simulink model "ModelMotS_dq_V2bis_FVC"  (R2019b)
settings: Solver=ode45  StartTime=0.0  StopTime=10  MaxStep=1e-4  RelTol=1e-4  EnableMultiTasking=on
undefined symbols (not defined in the file): Data_Ts, DiscIntNeverNeededParam, Inom, J, Jm, Lfr, Lfs, Lm, Lmt, Lr, Ls, np, P1, P2, Prdnom, Prinit, Psinit, Rr, Rs, SFC_Coeff, SLP_Coeff, thrinit, Tpwm, Vnom, wCurr, wCurr_PI, wL, wrinit, wSpeed_PI, wSpeedEst, xiCurr_PI, xiSpeed_PI
libraries: simulink x5
settings Model: Creator=stbp106  LastModifiedBy=versag
settings DataIOCC: LimitDataPoints=on  SaveFormat=Array  ReturnWorkspaceOutputs=off
settings OptimizationCC: LifeSpan=inf
settings DebuggingCC: UnderspecifiedInitializationDetection=Classic  MergeDetectMultiDrivingBlocksExec=none  SolverPrmCheckMsg=warning  SFUnexpectedBacktrackingDiag=warning  SFNoUnconditionalDefaultTransitionDiag=warning  SFExecutionAtInitializationDiag=none  ArithmeticOperatorsInVariantConditions=warning
settings HardwareCC: ProdBitPerPointer=32  ProdBitPerSizeT=32  ProdBitPerPtrDiffT=32  ProdLargestAtomicFloat=None  ProdIntDivRoundTo=Undefined  ProdEndianess=Unspecified  ProdWordSize=32  ProdHWDeviceType=32-bit Generic
settings ModelReferenceCC: PropagateSignalLabelsOutOfModel=off
settings SFSimCC: SimUseLocalCustomCode=off  CustomCodeUndefinedFunction=UseInterfaceOnly
settings RTWCC: RTWUseLocalCustomCode=off
settings CodeAppCC: StateflowObjectComments=on
settings GRTTargetCC: TargetLangStandard=C89/C90 (ANSI)  GeneratePreprocessorConditionals=Disable all
settings ConfigComp: CovMetricSettings=dw  CovHtmlReporting=on  CovSaveCumulativeToWorkspaceVar=on  CovSaveSingleToWorkspaceVar=on  CovExternalEMLEnable=off  CovSFcnEnable=off

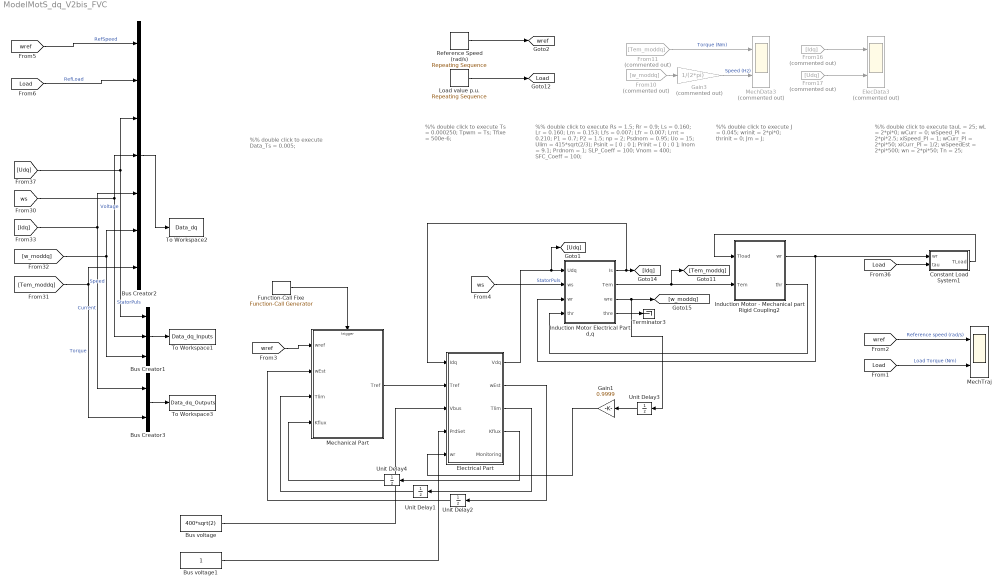
== system ModelMotS_dq_V2bis_FVC ==
  note: %% double click to execute
      |
      | Rs = 1.5; Rr = 0.9;
      | Ls = 0.160; Lr = 0.160; Lm = 0.153;
      | Lfs = 0.007; Lfr = 0.007; Lmt = 0.210; P1 = 0.7; P2 = 1.5;
      | np = 2;
      | Psdnom = 0.95; Uo = 15; Ulim = 415*sqrt(2/3);
      | Psinit = [ 0 ; 0 ]; Prinit = [ 0 ; 0 ];
      | Inom = 9.1; Prdnom = 1; SLP_Coeff = 100; Vnom = 400;
      | SFC_Coeff = 100;
  note: %% double click to execute
      |
      | J = 0.045;
      | wrinit = 2*pi*0;
      | thrinit = 0;
      | Jm = J;
  note: %% double click to execute
      |
      | tauL = 25;
      | wL = 2*pi*0;
      |
      | wCurr = 0;
      | wSpeed_PI = 2*pi*2.5; xiSpeed_PI = 1;
      | wCurr_PI = 2*pi*50; xiCurr_PI = 1/2;
      | wSpeedEst = 2*pi*500;
      |
      | wn = 2*pi*50;
      | Tn = 25;
  note: %% double click to execute
      |
      | Ts = 0.000250;
      | Tpwm = Ts;
      | Tfixe = 500e-6;
  note: %% double click to execute
      |
      | Data_Ts = 0.005;
  Bus Creator1 : BusCreator  Inputs=3
  Bus Creator2 : BusCreator  Inputs=7
  Bus Creator3 : BusCreator  Inputs=2
  Bus voltage : Constant  Value=400*sqrt(2)
  Bus voltage1 : Constant
  Constant Load System1 : Subsystem  Description=""
  ElecData3 : Scope  Commented=on  NumInputPorts=2
  Electrical Part : Subsystem
  From10 : From  Commented=on  GotoTag=w_moddq
  From11 : From  Commented=on  GotoTag=Tem_moddq
  From16 : From  Commented=on  GotoTag=Idq
  From17 : From  Commented=on  GotoTag=Udq
  Function-Call Fixe : simulink/Ports & Subsystems/Function-Call Generator  sample_time=Tfixe  numberOfIterations=1
  Gain1 : Gain  Gain=0.9999
  Gain3 : Gain  Commented=on  Gain=1/(2*pi)  SaturateOnIntegerOverflow=on  OutDataTypeStr=Inherit: Same as input  ParamDataTypeStr=Inherit: Same as input
  Induction Motor Electrical Part d,q : Subsystem  Description=""
  Induction Motor - Mechanical part Rigid Coupling2 : Subsystem  Description=""
  Load value p.u. : simulink/Sources/Repeating Sequence  rep_seq_t=[0 1 2.5 4 5.5 7 8.5 10]  rep_seq_y=[0 0 0 0 0 0 0 0] / 100 * 25
  MechData3 : Scope  Commented=on  NumInputPorts=2
  MechTraj : Scope  NumInputPorts=2
  Mechanical Part : Subsystem
  Reference Speed (rad/s) : simulink/Sources/Repeating Sequence  rep_seq_t=[0 1 2.5 4 5.5 7 8.5 10]  rep_seq_y=[0 0 50 50 -50 -50 25 25]*2*pi
  Terminator3 : Terminator
  To Workspace1 : ToWorkspace  VariableName=Data_dq_Inputs  SaveFormat=Timeseries  SampleTime=Data_Ts
  To Workspace2 : ToWorkspace  VariableName=Data_dq  SaveFormat=Timeseries  SampleTime=Data_Ts
  To Workspace3 : ToWorkspace  VariableName=Data_dq_Outputs  SaveFormat=Timeseries  SampleTime=Data_Ts
  Unit Delay{1..4} (4 alike) : UnitDelay  SampleTime=-1  HasFrameUpgradeWarning=on
  tag scope: Load=global, wref=global
  wires:
  Reference Speed (rad/s)/1 -> [wref]
  Induction Motor - Mechanical part Rigid Coupling2/2(thr) -> Induction Motor Electrical Part d,q/4(thr)
  Induction Motor Electrical Part d,q/2(Tem) -> [Tem_moddq], Induction Motor - Mechanical part Rigid Coupling2/2(Tem)
  Induction Motor - Mechanical part Rigid Coupling2/1(wr) -> Constant Load System1/1(wr), Induction Motor Electrical Part d,q/3(wr)
  Induction Motor Electrical Part d,q/4(thre) -> Terminator3/1
  Constant Load System1/1(TLoad) -> Induction Motor - Mechanical part Rigid Coupling2/1(Tload)
  Induction Motor Electrical Part d,q/1(Is) -> Electrical Part/1(Idq), [Idq]
  Induction Motor Electrical Part d,q/3(wre) -> Unit Delay3/1, [w_moddq]
  [Load] -> Constant Load System1/2(tau)
  From16/1 -> ElecData3/1
  From17/1 -> ElecData3/2
  From10/1 -> Gain3/1
  From11/1 -> MechData3/1  "Torque (Nm)"
  Gain3/1 -> MechData3/2  "Speed (Hz)"
  Load value p.u./1 -> [Load]
  [Udq] -> Bus Creator1/1, Bus Creator2/3  "Voltage"
  [Idq] -> Bus Creator3/1, Bus Creator2/5  "Current"
  [w_moddq] -> Bus Creator1/3, Bus Creator2/6  "Speed"
  [Tem_moddq] -> Bus Creator3/2, Bus Creator2/7  "Torque"
  Bus Creator2/1 -> To Workspace2/1
  [ws] -> Bus Creator1/2, Bus Creator2/4  "StatorPuls"
  [Load] -> MechTraj/2  "Load Torque (Nm)"
  [wref] -> MechTraj/1  "Reference speed (rad/s)"
  Mechanical Part/1(Tref) -> Electrical Part/2(Tref)
  [wref] -> Mechanical Part/1(wref)
  Electrical Part/2(wEst) -> Unit Delay2/1
  Electrical Part/3(Tlim) -> Unit Delay1/1
  Electrical Part/4(Kflux) -> Unit Delay4/1
  Unit Delay4/1 -> Mechanical Part/4(Kflux)
  Unit Delay1/1 -> Mechanical Part/3(Tlim)
  Unit Delay2/1 -> Mechanical Part/2(wEst)
  Electrical Part/1(Vdq) -> [Udq], Induction Motor Electrical Part d,q/1(Udq)
  [ws] -> Induction Motor Electrical Part d,q/2(ws)  "StatorPuls"
  Unit Delay3/1 -> Gain1/1
  Gain1/1 -> Electrical Part/5(wr)
  Bus voltage/1 -> Electrical Part/3(Vbus)
  Bus voltage1/1 -> Electrical Part/4(PrdSet)
  Function-Call Fixe/1 -> Mechanical Part/Trigger
  Bus Creator3/1 -> To Workspace3/1
  Bus Creator1/1 -> To Workspace1/1
  [wref] -> Bus Creator2/1  "RefSpeed"
  [Load] -> Bus Creator2/2  "RefLoad"

== system ModelMotS_dq_V2bis_FVC/Constant Load System1 ==
  wr : Inport
  tau : Inport  Port=2
  Constant1 : Constant  Value=wL
  Fcn : Fcn  Expr=u(1)/sqrt( u(1)^2 + (2*pi*0.1)^2)
  Product2 : Product  RndMeth=Zero
  Sum2 : Sum  Inputs=+-  SaturateOnIntegerOverflow=on  InputSameDT=on  OutDataTypeStr=Inherit: Same as first input
  TLoad : Outport  VectorParamsAs1DForOutWhenUnconnected=off
  wires:
  Product2/1 -> TLoad/1
  wr/1 -> Sum2/1
  Constant1/1 -> Sum2/2
  Sum2/1 -> Fcn/1
  Fcn/1 -> Product2/1
  tau/1 -> Product2/2

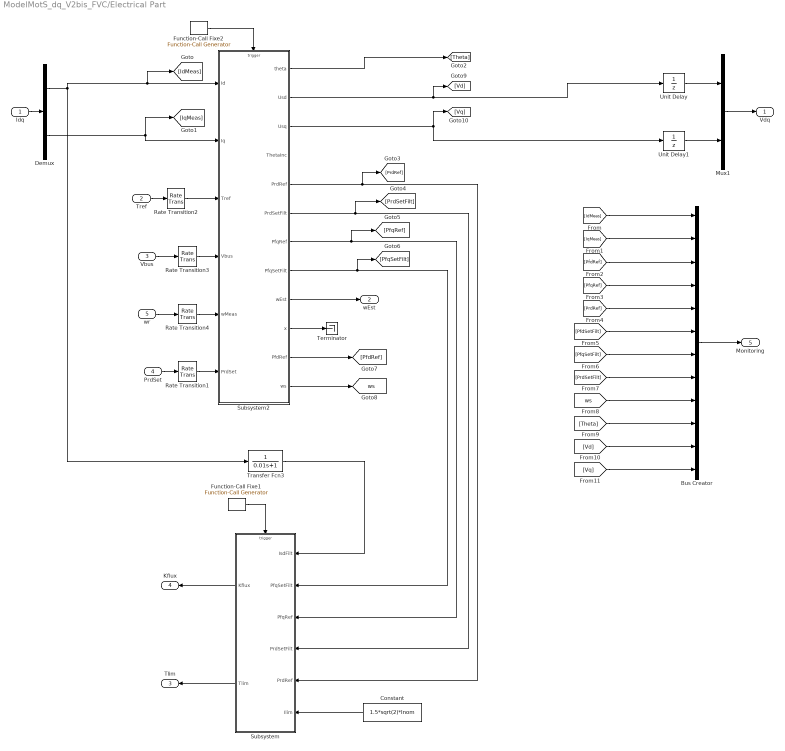
== system ModelMotS_dq_V2bis_FVC/Electrical Part ==
  Idq : Inport
  Tref : Inport  Port=2
  Vbus : Inport  Port=3
  PrdSet : Inport  Port=4
  wr : Inport  Port=5
  Bus Creator : BusCreator  Inputs=12
  Constant : Constant  Value=1.5*sqrt(2)*Inom
  Demux : Demux  Outputs=2
  Function-Call Fixe1 : simulink/Ports & Subsystems/Function-Call Generator  sample_time=Ts  numberOfIterations=1
  Function-Call Fixe2 : simulink/Ports & Subsystems/Function-Call Generator  sample_time=Ts  numberOfIterations=1
  Mux1 : Mux  Inputs=2
  Rate Transition{1..4} (4 alike) : RateTransition
  Subsystem : Subsystem
  Subsystem2 : Subsystem
  Terminator : Terminator
  Transfer Fcn3 : TransferFcn  Denominator=[0.01 1]
  Unit Delay : UnitDelay  SampleTime=-1  HasFrameUpgradeWarning=on
  Unit Delay1 : UnitDelay  SampleTime=-1  HasFrameUpgradeWarning=on
  Vdq : Outport  VectorParamsAs1DForOutWhenUnconnected=off
  wEst : Outport  Port=2  VectorParamsAs1DForOutWhenUnconnected=off
  Tlim : Outport  Port=3  VectorParamsAs1DForOutWhenUnconnected=off
  Kflux : Outport  Port=4  VectorParamsAs1DForOutWhenUnconnected=off
  Monitoring : Outport  Port=5  VectorParamsAs1DForOutWhenUnconnected=off
  tag scope: ws=global
  wires:
  [IqMeas] -> Bus Creator/2
  [IdMeas] -> Bus Creator/1
  [PfdRef] -> Bus Creator/3
  [PfqRef] -> Bus Creator/4
  [PrdRef] -> Bus Creator/5
  [PrdSetFilt] -> Bus Creator/8
  [PfqSetFilt] -> Bus Creator/7
  [PfdSetFilt] -> Bus Creator/6
  [ws] -> Bus Creator/9
  [Theta] -> Bus Creator/10
  Bus Creator/1 -> Monitoring/1
  Transfer Fcn3/1 -> Subsystem/1(IsdFilt)
  Subsystem/1(Kflux) -> Kflux/1
  Subsystem/2(Tlim) -> Tlim/1
  [Vd] -> Bus Creator/11
  [Vq] -> Bus Creator/12
  Subsystem2/7(PfqRef) -> [PfqRef], Subsystem/3(PfqRef)
  Subsystem2/6(PrdSetFilt) -> [PrdSetFilt], Subsystem/4(PrdSetFilt)
  Subsystem2/8(PfqSetFilt) -> [PfqSetFilt], Subsystem/2(PfqSetFilt)
  Subsystem2/1(theta) -> [Theta]
  Subsystem2/5(PrdRef) -> [PrdRef], Subsystem/5(PrdRef)
  Tref/1 -> Rate Transition2/1
  Vbus/1 -> Rate Transition3/1
  wr/1 -> Rate Transition4/1
  Subsystem2/9(wEst) -> wEst/1
  Subsystem2/11(PfdRef) -> [PfdRef]
  Subsystem2/12(ws) -> [ws]
  Demux/2 -> [IqMeas], Subsystem2/2(Iq)
  Demux/1 -> Subsystem2/1(Id), [IdMeas], Transfer Fcn3/1
  Function-Call Fixe2/1 -> Subsystem2/Trigger
  Function-Call Fixe1/1 -> Subsystem/Trigger
  Rate Transition2/1 -> Subsystem2/3(Tref)
  Subsystem2/10(x) -> Terminator/1
  Constant/1 -> Subsystem/6(Ilim)
  Rate Transition3/1 -> Subsystem2/4(Vbus)
  Rate Transition4/1 -> Subsystem2/5(wMeas)
  Mux1/1 -> Vdq/1
  PrdSet/1 -> Rate Transition1/1
  Rate Transition1/1 -> Subsystem2/6(PrdSet)
  Subsystem2/3(Usq) -> Unit Delay1/1, [Vq]
  Subsystem2/2(Usd) -> Unit Delay/1, [Vd]
  Unit Delay/1 -> Mux1/1
  Unit Delay1/1 -> Mux1/2
  Idq/1 -> Demux/1

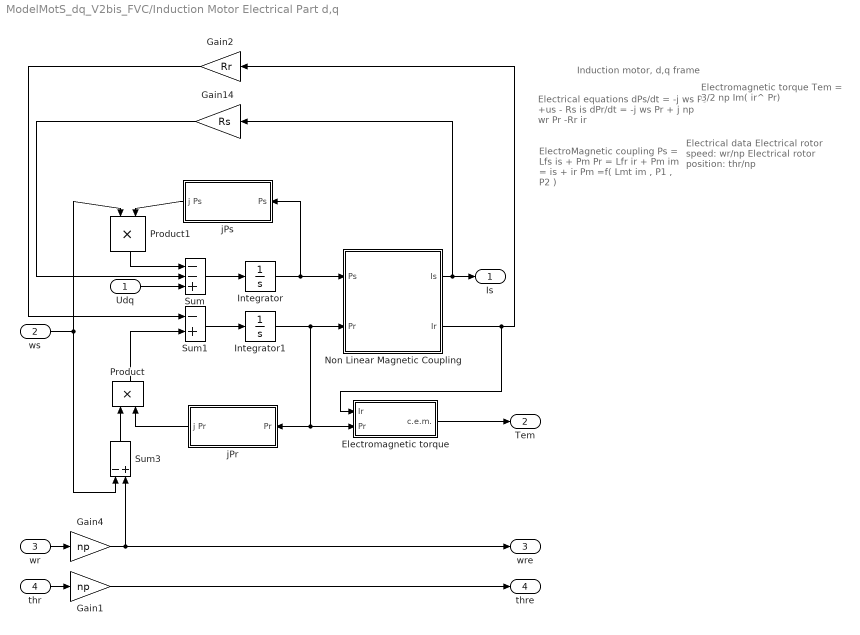
== system ModelMotS_dq_V2bis_FVC/Induction Motor Electrical Part d,q ==
  note: Electrical equations
      | dPs/dt =  -j ws Ps +us - Rs is
      | dPr/dt = -j ws Pr + j np wr Pr -Rr ir
  note: Electromagnetic torque
      | Tem = 3/2 np Im( ir^ Pr)
  note: Induction motor, d,q frame
  note: Electrical data
      | Electrical rotor speed: wr/np
      | Electrical rotor position: thr/np
  note: ElectroMagnetic coupling
      | Ps  = Lfs is + Pm
      | Pr  = Lfr ir + Pm
      |
      | im = is + ir
      | Pm =f( Lmt im , P1 , P2 )
  Udq : Inport
  ws : Inport  Port=2
  wr : Inport  Port=3
  thr : Inport  Port=4
  Electromagnetic torque : Subsystem
  Gain1 : Gain  Gain=np  SaturateOnIntegerOverflow=on  OutDataTypeStr=Inherit: Same as input  ParamDataTypeStr=Inherit: Same as input
  Gain14 : Gain  Gain=Rs  SaturateOnIntegerOverflow=on  OutDataTypeStr=Inherit: Same as input  ParamDataTypeStr=Inherit: Same as input
  Gain2 : Gain  Gain=Rr  SaturateOnIntegerOverflow=on  OutDataTypeStr=Inherit: Same as input  ParamDataTypeStr=Inherit: Same as input
  Gain4 : Gain  Gain=np  SaturateOnIntegerOverflow=on  OutDataTypeStr=Inherit: Same as input  ParamDataTypeStr=Inherit: Same as input
  Integrator : Integrator  InitialCondition=Psinit
  Integrator1 : Integrator  InitialCondition=Prinit
  Non Linear Magnetic Coupling : Subsystem
  Product : Product  SaturateOnIntegerOverflow=on  RndMeth=Zero  InputSameDT=on  OutDataTypeStr=Inherit: Same as first input
  Product1 : Product  SaturateOnIntegerOverflow=on  RndMeth=Zero  InputSameDT=on  OutDataTypeStr=Inherit: Same as first input
  Sum : Sum  Inputs=--+  SaturateOnIntegerOverflow=on  InputSameDT=on  OutDataTypeStr=Inherit: Same as first input
  Sum1 : Sum  Inputs=-+  SaturateOnIntegerOverflow=on  InputSameDT=on  OutDataTypeStr=Inherit: Same as first input
  Sum3 : Sum  Inputs=-+  SaturateOnIntegerOverflow=on  InputSameDT=on  OutDataTypeStr=Inherit: Same as first input
  jPr : Subsystem
  jPs : Subsystem
  Is : Outport  VectorParamsAs1DForOutWhenUnconnected=off
  Tem : Outport  Port=2  VectorParamsAs1DForOutWhenUnconnected=off
  wre : Outport  Port=3  VectorParamsAs1DForOutWhenUnconnected=off
  thre : Outport  Port=4  VectorParamsAs1DForOutWhenUnconnected=off
  wires:
  Integrator1/1 -> Non Linear Magnetic Coupling/2(Pr), Electromagnetic torque/2(Pr), jPr/1(Pr)
  Electromagnetic torque/1(c.e.m.) -> Tem/1
  Non Linear Magnetic Coupling/2(Ir) -> Electromagnetic torque/1(Ir), Gain2/1
  Product/1 -> Sum1/2
  jPr/1(j Pr) -> Product/2
  Gain2/1 -> Sum1/1
  Sum1/1 -> Integrator1/1
  Non Linear Magnetic Coupling/1(Is) -> Is/1, Gain14/1
  Sum/1 -> Integrator/1
  Udq/1 -> Sum/3
  Gain14/1 -> Sum/2
  jPs/1(j Ps) -> Product1/2
  Product1/1 -> Sum/1
  Integrator/1 -> Non Linear Magnetic Coupling/1(Ps), jPs/1(Ps)
  Sum3/1 -> Product/1
  Gain4/1 -> wre/1, Sum3/2
  ws/1 -> Product1/1, Sum3/1
  wr/1 -> Gain4/1
  thr/1 -> Gain1/1
  Gain1/1 -> thre/1

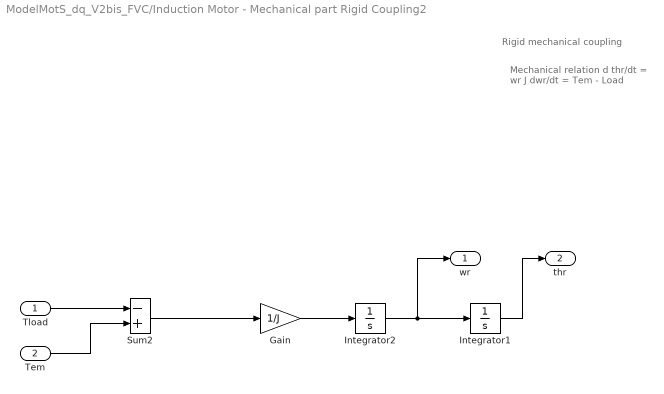
== system ModelMotS_dq_V2bis_FVC/Induction Motor - Mechanical part Rigid Coupling2 ==
  note: Rigid mechanical coupling
  note: Mechanical relation
      | d thr/dt = wr
      | J dwr/dt = Tem - Load
  Tload : Inport
  Tem : Inport  Port=2
  Gain : Gain  Gain=1/J  SaturateOnIntegerOverflow=on  OutDataTypeStr=Inherit: Same as input  ParamDataTypeStr=Inherit: Same as input
  Integrator1 : Integrator  InitialCondition=thrinit
  Integrator2 : Integrator  InitialCondition=wrinit
  Sum2 : Sum  Inputs=-+  SaturateOnIntegerOverflow=on  InputSameDT=on  OutDataTypeStr=Inherit: Same as first input
  wr : Outport  VectorParamsAs1DForOutWhenUnconnected=off
  thr : Outport  Port=2  VectorParamsAs1DForOutWhenUnconnected=off
  wires:
  Integrator1/1 -> thr/1
  Integrator2/1 -> wr/1, Integrator1/1
  Tem/1 -> Sum2/2
  Tload/1 -> Sum2/1
  Gain/1 -> Integrator2/1
  Sum2/1 -> Gain/1

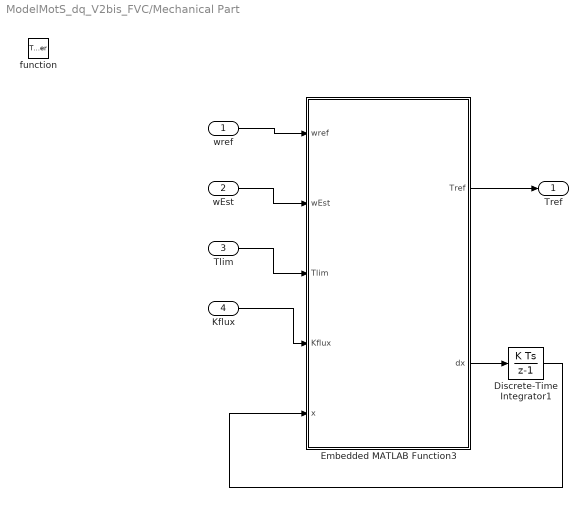
== system ModelMotS_dq_V2bis_FVC/Mechanical Part ==
  wref : Inport
  wEst : Inport  Port=2
  Tlim : Inport  Port=3
  Kflux : Inport  Port=4
  function : TriggerPort  TriggerType=function-call  VariantControl=(inherit)
  Discrete-Time Integrator1 : DiscreteIntegrator  InitialCondition=zeros(1,2)  SampleTime=-1  ICPrevOutput=DiscIntNeverNeededParam  ICPrevScaledInput=DiscIntNeverNeededParam
  Embedded MATLAB Function3 : MATLAB Function  TreatAsAtomicUnit=on
  Tref : Outport  VectorParamsAs1DForOutWhenUnconnected=off
  wires:
  Discrete-Time Integrator1/1 -> Embedded MATLAB Function3/5(x)
  wEst/1 -> Embedded MATLAB Function3/2(wEst)
  Tlim/1 -> Embedded MATLAB Function3/3(Tlim)
  wref/1 -> Embedded MATLAB Function3/1(wref)
  Embedded MATLAB Function3/2(dx) -> Discrete-Time Integrator1/1
  Embedded MATLAB Function3/1(Tref) -> Tref/1
  Kflux/1 -> Embedded MATLAB Function3/4(Kflux)

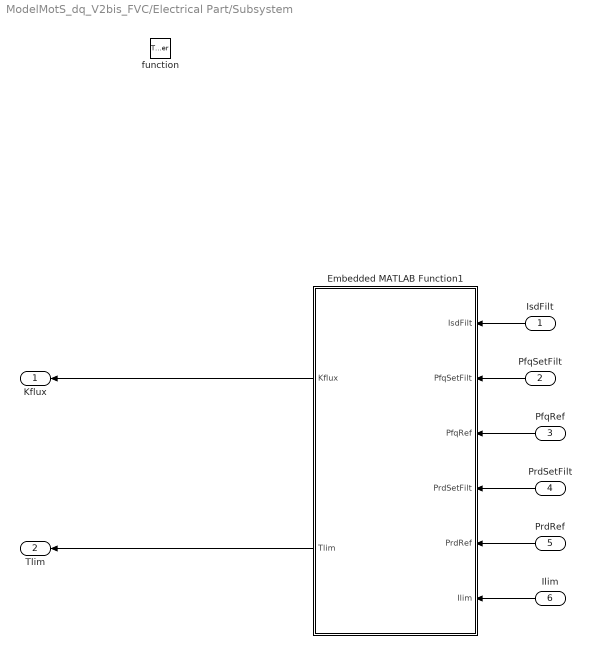
== system ModelMotS_dq_V2bis_FVC/Electrical Part/Subsystem ==
  IsdFilt : Inport
  PfqSetFilt : Inport  Port=2
  PfqRef : Inport  Port=3
  PrdSetFilt : Inport  Port=4
  PrdRef : Inport  Port=5
  Ilim : Inport  Port=6
  function : TriggerPort  TriggerType=function-call  VariantControl=(inherit)
  Embedded MATLAB Function1 : MATLAB Function  TreatAsAtomicUnit=on
  Kflux : Outport  VectorParamsAs1DForOutWhenUnconnected=off
  Tlim : Outport  Port=2  VectorParamsAs1DForOutWhenUnconnected=off
  wires:
  Embedded MATLAB Function1/2(Tlim) -> Tlim/1
  IsdFilt/1 -> Embedded MATLAB Function1/1(IsdFilt)
  Embedded MATLAB Function1/1(Kflux) -> Kflux/1
  PrdSetFilt/1 -> Embedded MATLAB Function1/4(PrdSetFilt)
  PfqSetFilt/1 -> Embedded MATLAB Function1/2(PfqSetFilt)
  PfqRef/1 -> Embedded MATLAB Function1/3(PfqRef)
  PrdRef/1 -> Embedded MATLAB Function1/5(PrdRef)
  Ilim/1 -> Embedded MATLAB Function1/6(Ilim)

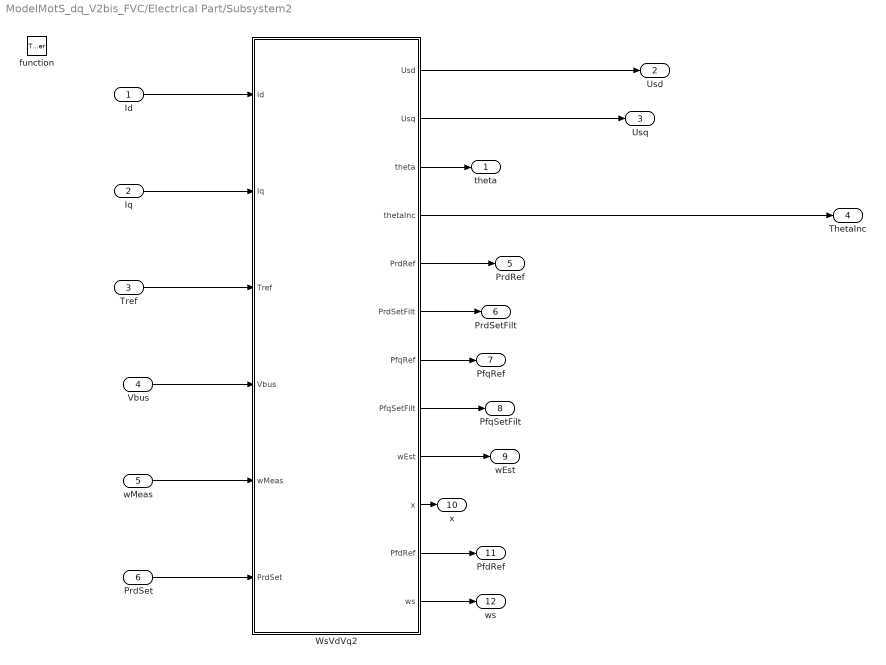
== system ModelMotS_dq_V2bis_FVC/Electrical Part/Subsystem2 ==
  Id : Inport
  Iq : Inport  Port=2
  Tref : Inport  Port=3
  Vbus : Inport  Port=4
  wMeas : Inport  Port=5
  PrdSet : Inport  Port=6
  function : TriggerPort  TriggerType=function-call  VariantControl=(inherit)
  WsVdVq2 : Subsystem
  theta : Outport  VectorParamsAs1DForOutWhenUnconnected=off
  Usd : Outport  Port=2  VectorParamsAs1DForOutWhenUnconnected=off
  Usq : Outport  Port=3  VectorParamsAs1DForOutWhenUnconnected=off
  ThetaInc : Outport  Port=4  VectorParamsAs1DForOutWhenUnconnected=off
  PrdRef : Outport  Port=5  VectorParamsAs1DForOutWhenUnconnected=off
  PrdSetFilt : Outport  Port=6  VectorParamsAs1DForOutWhenUnconnected=off
  PfqRef : Outport  Port=7  VectorParamsAs1DForOutWhenUnconnected=off
  PfqSetFilt : Outport  Port=8  VectorParamsAs1DForOutWhenUnconnected=off
  wEst : Outport  Port=9  VectorParamsAs1DForOutWhenUnconnected=off
  x : Outport  Port=10  VectorParamsAs1DForOutWhenUnconnected=off
  PfdRef : Outport  Port=11  VectorParamsAs1DForOutWhenUnconnected=off
  ws : Outport  Port=12  VectorParamsAs1DForOutWhenUnconnected=off
  wires:
  WsVdVq2/7(PfqRef) -> PfqRef/1
  WsVdVq2/9(wEst) -> wEst/1
  Tref/1 -> WsVdVq2/3(Tref)
  WsVdVq2/8(PfqSetFilt) -> PfqSetFilt/1
  WsVdVq2/6(PrdSetFilt) -> PrdSetFilt/1
  Vbus/1 -> WsVdVq2/4(Vbus)
  wMeas/1 -> WsVdVq2/5(wMeas)
  WsVdVq2/5(PrdRef) -> PrdRef/1
  WsVdVq2/3(theta) -> theta/1
  WsVdVq2/12(ws) -> ws/1
  WsVdVq2/11(PfdRef) -> PfdRef/1
  WsVdVq2/2(Usq) -> Usq/1
  WsVdVq2/4(thetaInc) -> ThetaInc/1
  WsVdVq2/1(Usd) -> Usd/1
  WsVdVq2/10(x) -> x/1
  Id/1 -> WsVdVq2/1(Id)
  Iq/1 -> WsVdVq2/2(Iq)
  PrdSet/1 -> WsVdVq2/6(PrdSet)

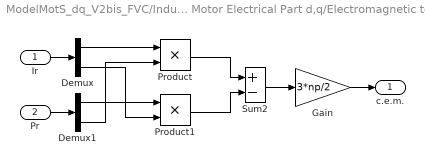
== system ModelMotS_dq_V2bis_FVC/Induction Motor Electrical Part d,q/Electromagnetic torque ==
  Ir : Inport
  Pr : Inport  Port=2
  Demux : Demux  Outputs=2
  Demux1 : Demux  Outputs=2
  Gain : Gain  Gain=3*np/2  SaturateOnIntegerOverflow=on  OutDataTypeStr=Inherit: Same as input  ParamDataTypeStr=Inherit: Same as input
  Product : Product  SaturateOnIntegerOverflow=on  RndMeth=Zero  InputSameDT=on  OutDataTypeStr=Inherit: Same as first input
  Product1 : Product  SaturateOnIntegerOverflow=on  RndMeth=Zero  InputSameDT=on  OutDataTypeStr=Inherit: Same as first input
  Sum2 : Sum  Inputs=+-  SaturateOnIntegerOverflow=on  InputSameDT=on  OutDataTypeStr=Inherit: Same as first input
  c.e.m. : Outport  VectorParamsAs1DForOutWhenUnconnected=off
  wires:
  Pr/1 -> Demux1/1
  Gain/1 -> c.e.m./1
  Ir/1 -> Demux/1
  Demux/2 -> Product1/2
  Demux1/1 -> Product1/1
  Demux1/2 -> Product/2
  Demux/1 -> Product/1
  Sum2/1 -> Gain/1
  Product1/1 -> Sum2/2
  Product/1 -> Sum2/1

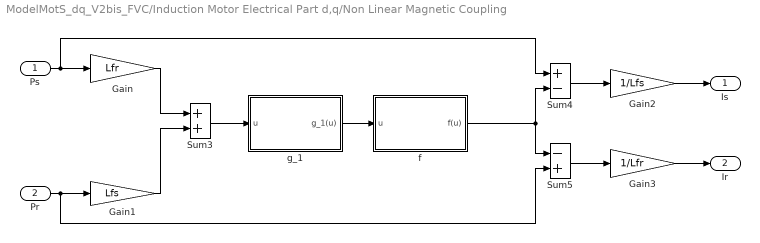
== system ModelMotS_dq_V2bis_FVC/Induction Motor Electrical Part d,q/Non Linear Magnetic Coupling ==
  Ps : Inport
  Pr : Inport  Port=2
  Gain : Gain  Gain=Lfr  SaturateOnIntegerOverflow=on  OutDataTypeStr=Inherit: Same as input  ParamDataTypeStr=Inherit: Same as input
  Gain1 : Gain  Gain=Lfs  SaturateOnIntegerOverflow=on  OutDataTypeStr=Inherit: Same as input  ParamDataTypeStr=Inherit: Same as input
  Gain2 : Gain  Gain=1/Lfs  SaturateOnIntegerOverflow=on  OutDataTypeStr=Inherit: Same as input  ParamDataTypeStr=Inherit: Same as input
  Gain3 : Gain  Gain=1/Lfr  SaturateOnIntegerOverflow=on  OutDataTypeStr=Inherit: Same as input  ParamDataTypeStr=Inherit: Same as input
  Sum3 : Sum  SaturateOnIntegerOverflow=on  InputSameDT=on  OutDataTypeStr=Inherit: Same as first input
  Sum4 : Sum  Inputs=+-  SaturateOnIntegerOverflow=on  InputSameDT=on  OutDataTypeStr=Inherit: Same as first input
  Sum5 : Sum  Inputs=-+  SaturateOnIntegerOverflow=on  InputSameDT=on  OutDataTypeStr=Inherit: Same as first input
  f : Subsystem
  g_1 : Subsystem
  Is : Outport  VectorParamsAs1DForOutWhenUnconnected=off
  Ir : Outport  Port=2  VectorParamsAs1DForOutWhenUnconnected=off
  wires:
  Gain2/1 -> Is/1
  Gain3/1 -> Ir/1
  Sum5/1 -> Gain3/1
  Sum4/1 -> Gain2/1
  Pr/1 -> Sum5/2, Gain1/1
  Ps/1 -> Sum4/1, Gain/1
  f/1(f(u)) -> Sum4/2, Sum5/1
  g_1/1(g_1(u)) -> f/1(u)
  Sum3/1 -> g_1/1(u)
  Gain1/1 -> Sum3/2
  Gain/1 -> Sum3/1

== system ModelMotS_dq_V2bis_FVC/Induction Motor Electrical Part d,q/jPr ==
  Pr : Inport
  Demux1 : Demux  Outputs=2
  Gain : Gain  Gain=-1  SaturateOnIntegerOverflow=on  OutDataTypeStr=Inherit: Same as input  ParamDataTypeStr=Inherit: Same as input
  Mux : Mux  Inputs=2
  j Pr : Outport  VectorParamsAs1DForOutWhenUnconnected=off
  wires:
  Mux/1 -> j Pr/1
  Gain/1 -> Mux/1
  Demux1/2 -> Gain/1
  Demux1/1 -> Mux/2
  Pr/1 -> Demux1/1

== system ModelMotS_dq_V2bis_FVC/Induction Motor Electrical Part d,q/jPs ==
  Ps : Inport
  Demux1 : Demux  Outputs=2
  Gain : Gain  Gain=-1  SaturateOnIntegerOverflow=on  OutDataTypeStr=Inherit: Same as input  ParamDataTypeStr=Inherit: Same as input
  Mux : Mux  Inputs=2
  j Ps : Outport  VectorParamsAs1DForOutWhenUnconnected=off
  wires:
  Ps/1 -> Demux1/1
  Demux1/1 -> Mux/2
  Demux1/2 -> Gain/1
  Gain/1 -> Mux/1
  Mux/1 -> j Ps/1

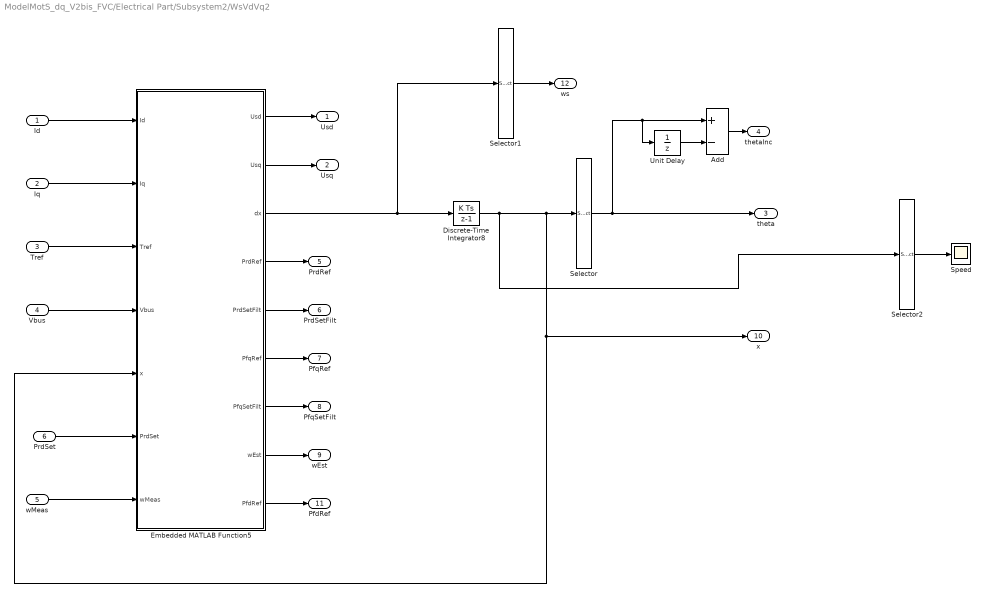
== system ModelMotS_dq_V2bis_FVC/Electrical Part/Subsystem2/WsVdVq2 ==
  Id : Inport
  Iq : Inport  Port=2
  Tref : Inport  Port=3
  Vbus : Inport  Port=4
  wMeas : Inport  Port=5
  PrdSet : Inport  Port=6
  Add : Sum  Inputs=+-
  Discrete-Time Integrator8 : DiscreteIntegrator  InitialCondition=[1/(Lm^2/Lr),0,1,zeros(1,9)]  SampleTime=-1  ICPrevOutput=DiscIntNeverNeededParam  ICPrevScaledInput=DiscIntNeverNeededParam
  Embedded MATLAB Function5 : MATLAB Function  TreatAsAtomicUnit=on
  Selector : Selector  InputPortWidth=12  IndexOptions=Index vector (dialog)  Indices=5  OutputSizes=1
  Selector1 : Selector  InputPortWidth=12  IndexOptions=Index vector (dialog)  Indices=5  OutputSizes=1
  Selector2 : Selector  InputPortWidth=12  IndexOptions=Index vector (dialog)  Indices=[11 12]  OutputSizes=1
  Speed : Scope
  Unit Delay : UnitDelay  SampleTime=-1  HasFrameUpgradeWarning=on
  Usd : Outport  VectorParamsAs1DForOutWhenUnconnected=off
  Usq : Outport  Port=2  VectorParamsAs1DForOutWhenUnconnected=off
  theta : Outport  Port=3  InitialOutput=[0]  VectorParamsAs1DForOutWhenUnconnected=off
  thetaInc : Outport  Port=4  InitialOutput=[0]  VectorParamsAs1DForOutWhenUnconnected=off
  PrdRef : Outport  Port=5  VectorParamsAs1DForOutWhenUnconnected=off
  PrdSetFilt : Outport  Port=6  VectorParamsAs1DForOutWhenUnconnected=off
  PfqRef : Outport  Port=7  VectorParamsAs1DForOutWhenUnconnected=off
  PfqSetFilt : Outport  Port=8  VectorParamsAs1DForOutWhenUnconnected=off
  wEst : Outport  Port=9  VectorParamsAs1DForOutWhenUnconnected=off
  x : Outport  Port=10  InitialOutput=[0]  VectorParamsAs1DForOutWhenUnconnected=off
  PfdRef : Outport  Port=11  VectorParamsAs1DForOutWhenUnconnected=off
  ws : Outport  Port=12  InitialOutput=[0]  VectorParamsAs1DForOutWhenUnconnected=off
  wires:
  wMeas/1 -> Embedded MATLAB Function5/7(wMeas)
  Unit Delay/1 -> Add/2
  Selector/1 -> theta/1, Unit Delay/1, Add/1
  Add/1 -> thetaInc/1
  Embedded MATLAB Function5/7(PfqSetFilt) -> PfqSetFilt/1
  Embedded MATLAB Function5/6(PfqRef) -> PfqRef/1
  Embedded MATLAB Function5/5(PrdSetFilt) -> PrdSetFilt/1
  Discrete-Time Integrator8/1 -> Selector2/1, Embedded MATLAB Function5/5(x), x/1, Selector/1
  Id/1 -> Embedded MATLAB Function5/1(Id)
  Iq/1 -> Embedded MATLAB Function5/2(Iq)
  Embedded MATLAB Function5/1(Usd) -> Usd/1
  Tref/1 -> Embedded MATLAB Function5/3(Tref)
  Embedded MATLAB Function5/2(Usq) -> Usq/1
  Vbus/1 -> Embedded MATLAB Function5/4(Vbus)
  Embedded MATLAB Function5/4(PrdRef) -> PrdRef/1
  Embedded MATLAB Function5/8(wEst) -> wEst/1
  Embedded MATLAB Function5/9(PfdRef) -> PfdRef/1
  Selector1/1 -> ws/1
  Embedded MATLAB Function5/3(dx) -> Selector1/1, Discrete-Time Integrator8/1
  PrdSet/1 -> Embedded MATLAB Function5/6(PrdSet)
  Selector2/1 -> Speed/1

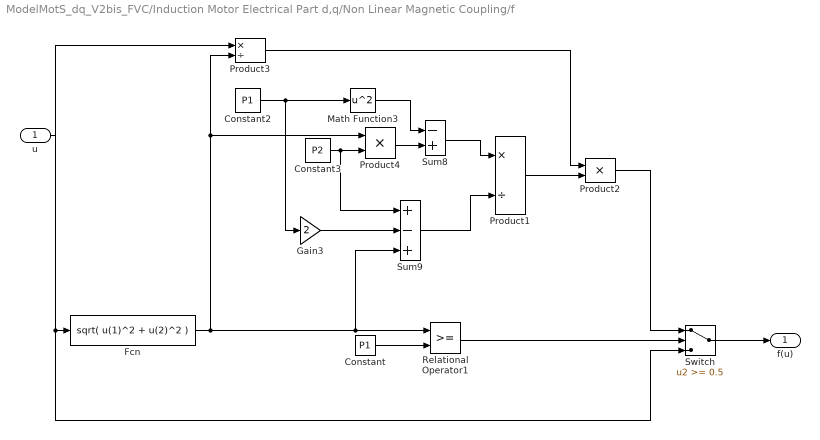
== system ModelMotS_dq_V2bis_FVC/Induction Motor Electrical Part d,q/Non Linear Magnetic Coupling/f ==
  u : Inport
  Constant : Constant  Value=P1
  Constant2 : Constant  Value=P1
  Constant3 : Constant  Value=P2
  Fcn : Fcn  Expr=sqrt( u(1)^2 + u(2)^2 )
  Gain3 : Gain  Gain=2  SaturateOnIntegerOverflow=on  OutDataTypeStr=Inherit: Same as input  ParamDataTypeStr=Inherit: Same as input
  Math Function3 : Math  Operator=square  SaturateOnIntegerOverflow=on
  Product1 : Product  Inputs=*/  SaturateOnIntegerOverflow=on  RndMeth=Zero  InputSameDT=on  OutDataTypeStr=Inherit: Same as first input
  Product2 : Product  SaturateOnIntegerOverflow=on  RndMeth=Zero  InputSameDT=on  OutDataTypeStr=Inherit: Same as first input
  Product3 : Product  Inputs=*/  SaturateOnIntegerOverflow=on  RndMeth=Zero  InputSameDT=on  OutDataTypeStr=Inherit: Same as first input
  Product4 : Product  SaturateOnIntegerOverflow=on  RndMeth=Zero  InputSameDT=on  OutDataTypeStr=Inherit: Same as first input
  Relational Operator1 : RelationalOperator  RndMeth=Nearest  InputSameDT=on
  Sum8 : Sum  Inputs=-+  SaturateOnIntegerOverflow=on  InputSameDT=on  OutDataTypeStr=Inherit: Same as first input
  Sum9 : Sum  Inputs=+-+  SaturateOnIntegerOverflow=on  InputSameDT=on  OutDataTypeStr=Inherit: Same as first input
  Switch : Switch  Threshold=0.5  SaturateOnIntegerOverflow=on  InputSameDT=on
  f(u) : Outport  InitialOutput=0  VectorParamsAs1DForOutWhenUnconnected=off
  wires:
  Fcn/1 -> Sum9/3, Relational Operator1/1, Product4/1, Product3/2
  Switch/1 -> f(u)/1
  Sum8/1 -> Product1/1
  Sum9/1 -> Product1/2
  Constant2/1 -> Gain3/1, Math Function3/1
  Gain3/1 -> Sum9/2
  Constant3/1 -> Sum9/1, Product4/2
  Math Function3/1 -> Sum8/1
  Product4/1 -> Sum8/2
  Product1/1 -> Product2/2
  Product3/1 -> Product2/1
  u/1 -> Switch/3, Fcn/1, Product3/1
  Relational Operator1/1 -> Switch/2
  Constant/1 -> Relational Operator1/2
  Product2/1 -> Switch/1

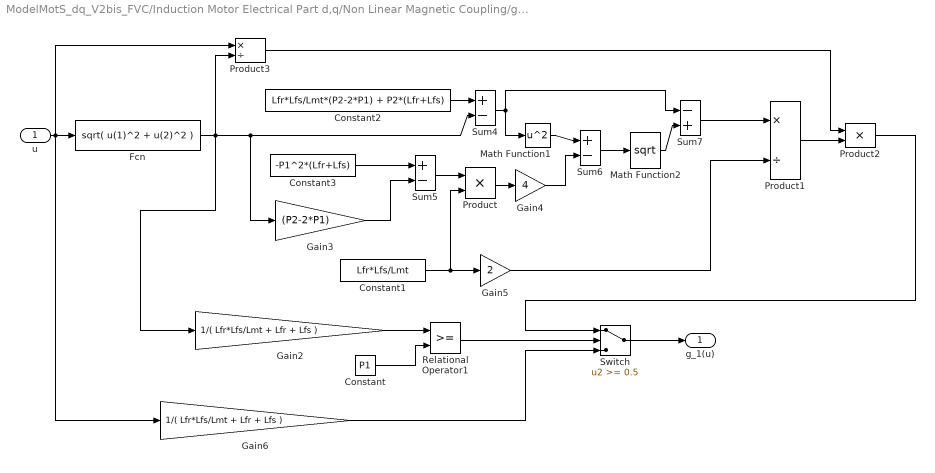
== system ModelMotS_dq_V2bis_FVC/Induction Motor Electrical Part d,q/Non Linear Magnetic Coupling/g_1 ==
  u : Inport
  Constant : Constant  Value=P1
  Constant1 : Constant  Value=Lfr*Lfs/Lmt
  Constant2 : Constant  Value=Lfr*Lfs/Lmt*(P2-2*P1) + P2*(Lfr+Lfs)
  Constant3 : Constant  Value=-P1^2*(Lfr+Lfs)
  Fcn : Fcn  Expr=sqrt( u(1)^2 + u(2)^2 )
  Gain2 : Gain  Gain=1/( Lfr*Lfs/Lmt + Lfr + Lfs )  SaturateOnIntegerOverflow=on  OutDataTypeStr=Inherit: Same as input  ParamDataTypeStr=Inherit: Same as input
  Gain3 : Gain  Gain=(P2-2*P1)  SaturateOnIntegerOverflow=on  OutDataTypeStr=Inherit: Same as input  ParamDataTypeStr=Inherit: Same as input
  Gain4 : Gain  Gain=4  SaturateOnIntegerOverflow=on  OutDataTypeStr=Inherit: Same as input  ParamDataTypeStr=Inherit: Same as input
  Gain5 : Gain  Gain=2  SaturateOnIntegerOverflow=on  OutDataTypeStr=Inherit: Same as input  ParamDataTypeStr=Inherit: Same as input
  Gain6 : Gain  Gain=1/( Lfr*Lfs/Lmt + Lfr + Lfs )  SaturateOnIntegerOverflow=on  OutDataTypeStr=Inherit: Same as input  ParamDataTypeStr=Inherit: Same as input
  Math Function1 : Math  Operator=square  SaturateOnIntegerOverflow=on
  Math Function2 : Math  Operator=sqrt  SaturateOnIntegerOverflow=on
  Product : Product  SaturateOnIntegerOverflow=on  RndMeth=Zero  InputSameDT=on  OutDataTypeStr=Inherit: Same as first input
  Product1 : Product  Inputs=*/  SaturateOnIntegerOverflow=on  RndMeth=Zero  InputSameDT=on  OutDataTypeStr=Inherit: Same as first input
  Product2 : Product  SaturateOnIntegerOverflow=on  RndMeth=Zero  InputSameDT=on  OutDataTypeStr=Inherit: Same as first input
  Product3 : Product  Inputs=*/  SaturateOnIntegerOverflow=on  RndMeth=Zero  InputSameDT=on  OutDataTypeStr=Inherit: Same as first input
  Relational Operator1 : RelationalOperator  RndMeth=Nearest  InputSameDT=on
  Sum4 : Sum  Inputs=+-  SaturateOnIntegerOverflow=on  InputSameDT=on  OutDataTypeStr=Inherit: Same as first input
  Sum5 : Sum  Inputs=+-  SaturateOnIntegerOverflow=on  InputSameDT=on  OutDataTypeStr=Inherit: Same as first input
  Sum6 : Sum  Inputs=+-  SaturateOnIntegerOverflow=on  InputSameDT=on  OutDataTypeStr=Inherit: Same as first input
  Sum7 : Sum  Inputs=-+  SaturateOnIntegerOverflow=on  InputSameDT=on  OutDataTypeStr=Inherit: Same as first input
  Switch : Switch  Threshold=0.5  SaturateOnIntegerOverflow=on  InputSameDT=on
  g_1(u) : Outport  InitialOutput=0  VectorParamsAs1DForOutWhenUnconnected=off
  wires:
  Switch/1 -> g_1(u)/1
  Gain6/1 -> Switch/3
  Product2/1 -> Switch/1
  Constant/1 -> Relational Operator1/2
  Gain2/1 -> Relational Operator1/1
  Relational Operator1/1 -> Switch/2
  u/1 -> Gain6/1, Product3/1, Fcn/1
  Product3/1 -> Product2/1
  Fcn/1 -> Gain2/1, Product3/2, Gain3/1, Sum4/2
  Constant1/1 -> Gain5/1, Product/2
  Sum5/1 -> Product/1
  Product/1 -> Gain4/1
  Product1/1 -> Product2/2
  Gain5/1 -> Product1/2
  Sum7/1 -> Product1/1
  Gain3/1 -> Sum5/2
  Constant3/1 -> Sum5/1
  Sum4/1 -> Sum7/1, Math Function1/1
  Math Function2/1 -> Sum7/2
  Sum6/1 -> Math Function2/1
  Math Function1/1 -> Sum6/1
  Constant2/1 -> Sum4/1
  Gain4/1 -> Sum6/2

== matlab function ModelMotS_dq_V2bis_FVC/Mechanical Part/Embedded MATLAB Function3 ==
  data: Tref output; dx output; wref input; wEst input; Tlim input; Kflux input; x input; wSpeed_PI parameter; xiSpeed_PI parameter; SFC_Coeff parameter; Jm parameter; np parameter
function [Tref, dx] = ControlLaw(wref, wEst,  Tlim, Kflux,x,wSpeed_PI,xiSpeed_PI,SFC_Coeff, Jm,np)
%#eml

%dx=[dwInputRef, dIsdSetFilt, dIsqSetFilt, ws, dwEst, dPfdE, dPfqE, dTint, dwd, dwq];


wInputRef=x(1);
Tint=x(2);

JmEst = Jm;

xi = xiSpeed_PI;
v0 = wSpeed_PI;
kp = JmEst/np*2*xi*v0;
ki = JmEst/np*v0^2; 

%%%%
%%%% Speed reference
%%%%                
   dwInputRef = ki/kp*( wref - wInputRef );   
   wInputRef2 = SFC_Coeff/100*wref + (1-SFC_Coeff/100)*wInputRef;
  
   wb = wEst;
   Tref = kp*(wInputRef2 - wb) + Tint;
   Trefbuf = Tref;
   if (abs(Tref)>Tlim) 
       Tref = sign(Tref)*Tlim; 
   end
   
   dTint = ( ki*(wInputRef2 - wb) + 1.5*ki/kp*(Tref - Trefbuf))*Kflux;
   
   dx=[dwInputRef, dTint];

== matlab function ModelMotS_dq_V2bis_FVC/Electrical Part/Subsystem/Embedded MATLAB Function1 ==
  data: Kflux output; Tlim output; IsdFilt input; PfqSetFilt input; PfqRef input; PrdSetFilt input; PrdRef input; Rs parameter; Rr parameter; Ls parameter; Lr parameter; Lm parameter; Jm parameter; np parameter; Inom parameter; Prdnom parameter; Ilim input
function [Kflux, Tlim] = ControlLaw(IsdFilt,PfqSetFilt,PfqRef,PrdSetFilt,PrdRef, Rs,Rr,Ls,Lr,Lm,Jm,np,Inom, Prdnom,Ilim)
%#eml

Lf = Ls - Lm^2/Lr; 
Tr = Lr/Rr; 
invTr = 1/Tr; 
Rreq = Rr*(Lm/Lr)^2; 
Req = Rs + Rreq; 
L = Lm^2/Lr;
JmEst = Jm;
sig=Lf/Ls;

LfEst = Lf;
LEst = L;
invTrEst = invTr;
RsEst = Rs;
RreqEst = Rreq;
sigEst = sig;

%Ilim = 1.5*sqrt(2)*Inom;

PrdSet=Prdnom;
%%%%
%%%% Current Limitation
%%%%
   if (PrdSetFilt<PrdSet/64) Kflux = 1; 
   else if (PrdRef<PrdSet/64) Kflux = 1; 
   else Kflux = (PrdRef/PrdSetFilt)^2; 
   end;
   end;
   
   if (PrdSetFilt>PrdSet/16) 
     Tnorm = 3/2*np*PrdSetFilt*PrdSet/LEst;
   else
     Tnorm = 3/2*np*(PrdSet/16)*PrdSet/LEst;  
   end
   
   IdBC = IsdFilt;
   if ( (IdBC>Ilim) || (IdBC<-Ilim) )
       Tlim = 0.
   else 
       minU = 1;
       if ((PfqSetFilt*PrdRef*PrdSetFilt)~=0) minU = (PfqRef/PfqSetFilt)/(PrdRef/PrdSetFilt); end;
       if (minU > 2.) minU = 2.; else if (minU < 1.) minU = 1.; end; end; 
       IlimTMP = Ilim;
       IsqLim = sqrt(IlimTMP^2-IdBC^2)/minU;
       Tlim = 3/2*np*PrdRef*IsqLim/Kflux;
   end

== matlab function ModelMotS_dq_V2bis_FVC/Electrical Part/Subsystem2/WsVdVq2/Embedded MATLAB Function5 ==
  data: Usd output; Usq output; Id input; dx output; Iq input; Tref input; Vbus input; x input; PrdSet input; Rs parameter; Rr parameter; Ls parameter; Lr parameter; Lm parameter; Jm parameter; np parameter; Vnom parameter; wCurr_PI parameter; xiCurr_PI parameter; Prdnom parameter; wCurr parameter; wSpeedEst parameter; PrdRef output; PrdSetFilt output; PfqRef output; PfqSetFilt output; wEst output; SLP_Coeff parameter; PfdRef output; Tpwm parameter; wMeas input
function [Usd, Usq, dx, PrdRef, PrdSetFilt, PfqRef, PfqSetFilt, wEst,PfdRef] = ControlLaw(Id,Iq,Tref,Vbus,x,PrdSet, Rs,Rr,Ls,Lr,Lm,Jm,np,Vnom,wCurr_PI,xiCurr_PI,Prdnom,wCurr,wSpeedEst,SLP_Coeff,Tpwm,wMeas)
%#eml

%   dx=[dIsdSetFilt, dIsqSetFilt, dPrdSetFilt, ws, dwEst, dPfdE, dPfqE, dPrdE, dwq];
IsdSetFilt=x(1);
IsqSetFilt=x(2);
PrdSetFilt=x(3);
PrqSetFilt=x(4);
Theta=x(5);
wEst=x(6);
PfdE=x(7);
PfqE=x(8);
PrdE=x(9);
PrqE=x(10);
wd=x(11);
wq=x(12);

Lf = Ls - Lm^2/Lr; 
Tr = Lr/Rr; 
invTr = 1/Tr; 
Rreq = Rr*(Lm/Lr)^2; 
Req = Rs + Rreq; 
L = Lm^2/Lr;
JmEst = Jm;
sig=Lf/Ls;

LfEst = Lf;
LEst = L;
invTrEst = invTr;
RsEst = Rs;
RreqEst = Rreq;
sigEst = sig;
ReqEst=RreqEst+RsEst;

vlim = Vbus/sqrt(3);

w1 = wCurr_PI;
w0 = 2*xiCurr_PI*w1;

PrdSet = Prdnom;
PfdSetFilt = LfEst*IsdSetFilt;
PfqSetFilt = LfEst*IsqSetFilt;
PfdRef = PfdE + PfdSetFilt;
PfqRef = PfqE + PfqSetFilt;
IsdRef = PfdRef/LfEst;
IsqRef = PfqRef/LfEst;
PrdRef = PrdE + PrdSetFilt ;
PrqRef = PrqE + PrqSetFilt ;

%%%%
%%%% Measure
%%%%

   IsdM = Id ;
   IsqM = Iq ;
   PfdM = LfEst*IsdM;
   PfqM = LfEst*IsqM;
   
%%%%
%%%% Set Point 
%%%%
   IPrdSet = PrdSet/LEst; 
   IsdSet = IPrdSet; 
   if (PrdSetFilt>PrdSet/16)
       IsqSet = (Tref/(3/2*np*PrdSetFilt));
       %IsqSet = (Tref/(3/2*np*PrdRef));
   else
       IsqSet = (Tref/(3/2*np*PrdSet/16));
   end
   
   PfdSet = LfEst*IsdSet; 
   PfqSet = LfEst*IsqSet;

%%%%
%%%% Set Point Filtering
%%%%

    if (wCurr==0)
        wCurr1 = (RsEst+RreqEst)/LfEst;
    else
        wCurr1=wCurr;
    end
        
   dIsdSetFilt = wCurr1*(IsdSet - IsdSetFilt) ;
   dIsqSetFilt = wCurr1*(IsqSet - IsqSetFilt);

   Pfdq = PfdM + 1j*PfqM;
   PfdqRef = PfdRef + 1j*PfqRef; 
   PrdqRef = PrdRef + 1j*PrqRef;  
   IdqRef = PfdqRef/LfEst;

   wo = sqrt( invTrEst^2 + wEst^2 );
   lam = (RreqEst/LfEst)/wo;

   corVrE = (-RreqEst/LfEst-lam*(invTrEst+1j*wEst))*( - 0.);
   corVr = (-RreqEst/LfEst-lam*(invTrEst+1j*wEst))*(Pfdq-PfdqRef) ;
   
   dPrdSetFilt = invTrEst*(PrdSet-PrdSetFilt) - real(corVr);
   dPrqSetFilt = 0;

   PfdSetFilt = LfEst*IsdSetFilt; 
   PfqSetFilt = LfEst*IsqSetFilt;

%%%%
%%%% Stator Frequency
%%%%               
   if (PrdRef>PrdSet/16)
     wgCor= (RreqEst/LfEst*PfqRef -imag(corVr))/PrdRef;
   else
     wgCor= (RreqEst/LfEst*PfqRef -imag(corVr))/(PrdSet/16);  
   end
   
   dwEst = wSpeedEst*(wMeas - wEst);
   ws   = wEst + SLP_Coeff*wgCor/100.0 ;

%%%%
%%%% Gain Calculation
%%%%                   
   tempwd = (PfdRef-PfdM)/Prdnom;
   dwd = w1*w1*tempwd;
   propwd = w0*tempwd;   wdInt = propwd + wd;    
      
   tempwq = (PfqRef-PfqM)/Prdnom;
   dwq = w1*w1*tempwq;
   propwq = w0*tempwq;   wqInt = propwq + wq;           


%
% Voltage Calculation
%                
%    UsdRef = (RsEst+RreqEst)/LfEst*PfdSetFilt + wCurr1*(PfdSet-PfdSetFilt) - ws*PfqSetFilt - invTrEst*PrdSetFilt + wdInt*Prdnom; 
%    UsqRef = ws*PfdSetFilt + (RsEst+RreqEst)/LfEst*PfqSetFilt + wCurr1*(PfqSet-PfqSetFilt)+ wEst*PrdSetFilt + wqInt*Prdnom; 
   UsdRef = (RsEst+RreqEst)/LfEst*PfdSetFilt + wCurr1*(PfdSet-PfdSetFilt) - ws*PfqSetFilt - invTrEst*PrdRef + wdInt*Prdnom; 
   UsqRef = ws*PfdSetFilt + (RsEst+RreqEst)/LfEst*PfqSetFilt + wCurr1*(PfqSet-PfqSetFilt)+ wEst*PrdRef + wqInt*Prdnom; 

   
   UsdqRef = sqrt( UsdRef^2+UsqRef^2);                   

%
% Voltage Limitation
%                
if (UsdqRef>vlim) 
   	Usd = UsdRef/UsdqRef*vlim; 
   	Usq = UsqRef/UsdqRef*vlim; 
else 
   Usd = UsdRef; Usq = UsqRef; 
end;

%
% FieldWeakening Calculation
%                
    Xd = Usd - UsdRef+ invTrEst*PrdE;
   Xq = Usq - UsqRef- wEst*PrdE; 
   
   Xd = Usd - UsdRef;%+ invTrEst*PrdE;
   Xq = Usq - UsqRef;%- wEst*PrdE; 
   Zd = (ReqEst/LfEst * Xd + ws * Xq)/(ReqEst^2/(LfEst*LfEst)+ws^2);
   Zq = (Req/LfEst * Xq - ws * Xd)/(ReqEst^2/(LfEst*LfEst)+ws^2);
   
   Bd = -PfdE + Zd;
   Bq = -PfqE + Zq;
   
   ThetaInc = ws*Tpwm;
   A11 = ((1-cos(ThetaInc))/Tpwm + cos(ThetaInc)*ReqEst/LfEst);
   A12 = (-sin(ThetaInc)/Tpwm + sin(ThetaInc)*ReqEst/LfEst);
   A21 = (sin(ThetaInc)/Tpwm - sin(ThetaInc)*ReqEst/LfEst);
   A22 = ((1-cos(ThetaInc))/Tpwm + cos(ThetaInc)*ReqEst/LfEst);
   
   dPfdE = A11*Bd + A12*Bq;
   dPfqE = A21*Bd + A22*Bq;
   
   dPrdE = (-invTrEst*PrdE + RreqEst/LfEst*PfdE );
   dPrqE = 0;   
   IsdE = PfdE/LfEst;
   IsqE = PfqE/LfEst;
   
   dx=[dIsdSetFilt; dIsqSetFilt; dPrdSetFilt;dPrqSetFilt; ws; dwEst; dPfdE; dPfqE; dPrdE;dPrqE; dwd; dwq];
